simulink model "nuri3s_computed_torque_uncertainty1"  (R2024b)
settings: Solver=VariableStepAuto  StartTime=0.0  StopTime=10  RelTol=1e-3
undefined symbols (not defined in the file): timepoints, waypoints
libraries: robotmaniplib x2, robotcorelib x1
settings Model: Creator=user  LastModifiedBy=변재형

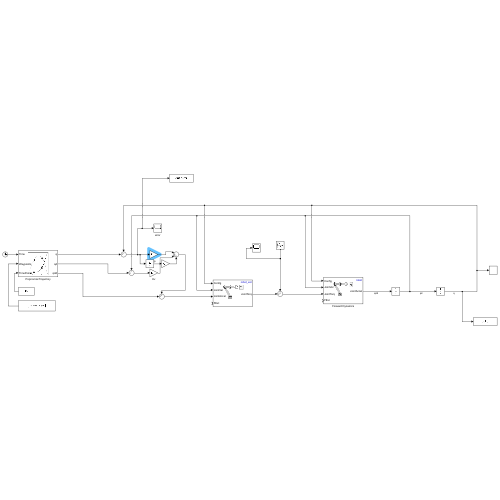
[thumbnail: Simulink's stored preview of the top-level diagram]
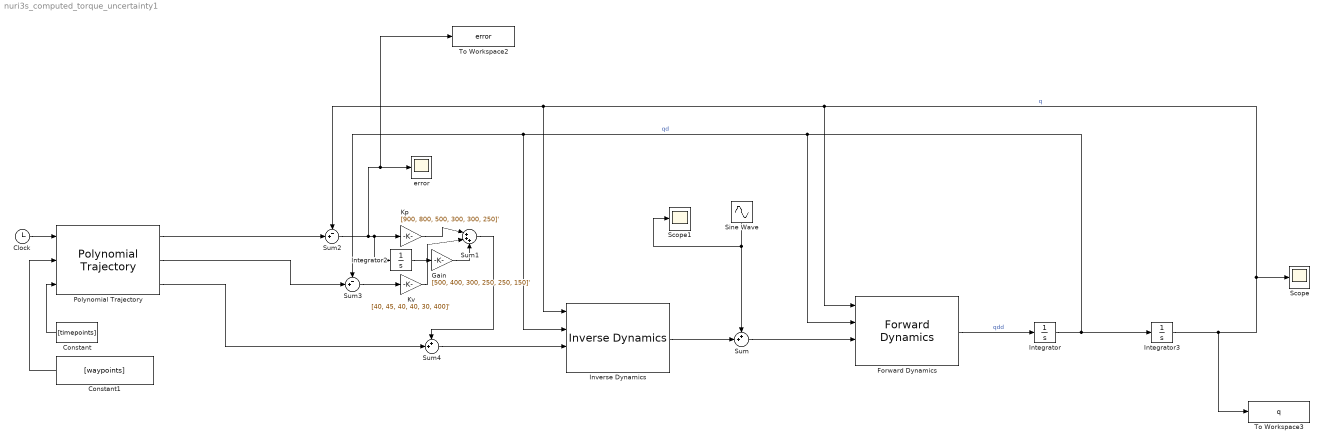
== system nuri3s_computed_torque_uncertainty1 ==
  Clock : Clock
  Constant : Constant  Value=[timepoints]
  Constant1 : Constant  Value=[waypoints]
  Forward Dynamics : robotmaniplib/Forward Dynamics  RigidBodyTree=robot  SimulateUsing=Interpreted execution
  Gain : Gain  Gain=[500, 400, 300, 250, 250, 150]'
  Integrator : Integrator  InitialCondition=[0 0 -1.57 0 -1.57 0]
  Integrator2 : Integrator
  Integrator3 : Integrator  InitialCondition=[0 0 -1.57 0 -1.57 0]
  Inverse Dynamics : robotmaniplib/Inverse Dynamics  RigidBodyTree=robot_est  SimulateUsing=Interpreted execution
  Kp : Gain  Gain=[900, 800, 500, 300, 300, 250]'
  Kv : Gain  Gain=[40, 45, 40, 40, 30, 400]'
  Polynomial Trajectory : robotcorelib/Polynomial Trajectory  WaypointSource=External  Waypoints=[ 0, 2, 1, 5, 0; -1, 3, 1, 4, 4 ]  TimePoints=[ 0, 1, 2, 3, 4 ]  TimeInterval=[ 1, 4 ]  Method=Quintic Polynomial  ParameterSource=Internal  VelocityBoundaryCondition=zeros( 6, 100)  AccelerationBoundaryCondition=zeros( 6, 100 )  SimulateUsing=Interpreted execution
  Scope : Scope
  Scope1 : Scope
  Sine Wave : Sin  Amplitude=0.1  Frequency=10  SampleTime=0
  Sum : Sum  Inputs=++|
  Sum1 : Sum  Inputs=|+++
  Sum2 : Sum  Inputs=-+|
  Sum3 : Sum  Inputs=-+|
  Sum4 : Sum  Inputs=++|
  To Workspace2 : ToWorkspace  VariableName=error  SaveFormat=Structure With Time  SampleTime=-1
  To Workspace3 : ToWorkspace  VariableName=q  SaveFormat=Structure With Time  SampleTime=-1
  error : Scope
  wires:
  Forward Dynamics/1 -> Integrator/1  "qdd"
  Integrator/1 -> Integrator3/1, Forward Dynamics/2, Inverse Dynamics/2, Sum3/1  "qd"
  Integrator3/1 -> To Workspace3/1, Scope/1, Forward Dynamics/1, Inverse Dynamics/1, Sum2/1  "q"
  Clock/1 -> Polynomial Trajectory/1
  Constant/1 -> Polynomial Trajectory/3
  Constant1/1 -> Polynomial Trajectory/2
  Kp/1 -> Sum1/1
  Sum3/1 -> Kv/1
  Sum2/1 -> Integrator2/1, Kp/1, To Workspace2/1, error/1
  Sum4/1 -> Inverse Dynamics/3
  Polynomial Trajectory/1 -> Sum2/2
  Polynomial Trajectory/2 -> Sum3/2
  Polynomial Trajectory/3 -> Sum4/2
  Sum1/1 -> Sum4/1
  Kv/1 -> Sum1/2
  Integrator2/1 -> Gain/1
  Gain/1 -> Sum1/3
  Inverse Dynamics/1 -> Sum/2
  Sum/1 -> Forward Dynamics/3
  Sine Wave/1 -> Scope1/1, Sum/1
